simulink model "wahadlo"  (R2021b)
settings: Solver=ode45  StartTime=0.0  StopTime=10.0  RelTol=1e-3  EnableMultiTasking=on
settings Model: Creator=Student  LastModifiedBy=adria
settings SolverCC: AlgebraicLoopSolver=TrustRegion
settings DataIOCC: LimitDataPoints=on  SaveFormat=Array  SignalLoggingSaveFormat=ModelDataLogs  ReturnWorkspaceOutputs=off  SignalLoggingName=sigsOut
settings OptimizationCC: ExpressionDepthLimit=2147483647  InitFltsAndDblsToZero=on  LifeSpan=inf
settings DebuggingCC: SaveWithParameterizedLinksMsg=none  UnderspecifiedInitializationDetection=Classic  MergeDetectMultiDrivingBlocksExec=none  SignalResolutionControl=TryResolveAllWithWarning  MultiTaskDSMMsg=warning  MultiTaskCondExecSysMsg=none  FcnCallInpInsideContextMsg=warning  StateNameClashWarn=warning  SFUnexpectedBacktrackingDiag=warning  SFNoUnconditionalDefaultTransitionDiag=warning  SFExecutionAtInitializationDiag=none  SFMachineParentedDataDiag=warning  ArithmeticOperatorsInVariantConditions=warning
settings HardwareCC: ProdBitPerPointer=32  ProdBitPerSizeT=32  ProdBitPerPtrDiffT=32  ProdLargestAtomicFloat=None  ProdIntDivRoundTo=Undefined  ProdEndianess=Unspecified  ProdWordSize=32  ProdHWDeviceType=32-bit Generic  TargetUnknown=on
settings ModelReferenceCC: PropagateSignalLabelsOutOfModel=off
settings SFSimCC: SimUseLocalCustomCode=off  CustomCodeUndefinedFunction=UseInterfaceOnly
settings RTWCC: RTWUseLocalCustomCode=off
settings CodeAppCC: StateflowObjectComments=on
settings GRTTargetCC: TargetFcnLib=ansi_tfl_tmw.mat  TargetLangStandard=C89/C90 (ANSI)  ModelReferenceCompliant=off  ParMdlRefBuildCompliant=off  CompOptLevelCompliant=off  ConcurrentExecutionCompliant=off  CombineOutputUpdateFcns=off  MatFileLogging=off  MATLABClassNameForMDSCustomization=Simulink.SoftwareTarget.TargetSpecificTriggerConfigurationBase  GRTInterface=on
settings ConfigComp: CovMetricSettings=dw  CovSaveCumulativeToWorkspaceVar=on  CovSaveSingleToWorkspaceVar=on  CovExternalEMLEnable=off

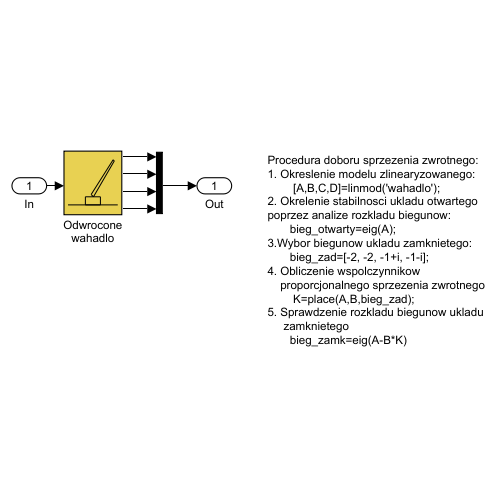
[thumbnail: Simulink's stored preview of the top-level diagram]
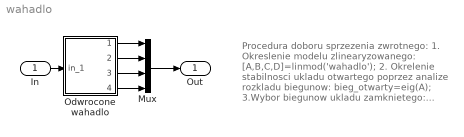
== system wahadlo ==
  note: Procedura doboru sprzezenia zwrotnego:
      | 1. Okreslenie modelu zlinearyzowanego:
      |         [A,B,C,D]=linmod('wahadlo');
      | 2. Okrelenie stabilnosci ukladu otwartego
      | poprzez analize rozkladu biegunow:
      |        bieg_otwarty=eig(A);
      | 3.Wybor biegunow ukladu zamknietego:
      |        bieg_zad=[-2, -2, -1+i, -1-i];
      | 4. Obliczenie wspolczynnikow
      |     proporcjonalnego sprzezenia zwrotnego
      |         K=place(A,B,bieg_zad);
      | 5. Sprawdzenie rozkladu biegunow ukladu
      |      zamknietego
      |        bieg_zamk=eig(A-B*K)
  In : Inport
  Mux : Mux
  Odwrocone wahadlo : Subsystem  mask(Odwrocone wahadlo){init_cond=[0  0  0  0], specs=[8         0.1           1         9.8]}
      mask prompts: init_cond "Poczatkowe(kat, predkosc katowa, pozycja wozka,  predkosc wozka):"; specs "Parametry (dlugosc, masa wahadla, masa wozka, g):"
      mask help: Odwrocone wahadlo
      mask init:
      | l=specs(1)/2;m=specs(2);mc=specs(3);g=specs(4);
      mask Help: Odwrocone wahadlo
      mask Display: plot(-4,-1,4,6,[0 3 2.8 -0.2 0],[1 5 5.15 1.15 1],[-1 -1 1 1 -1],[1 0 0 1 1],[-3.5 3.5],[0 0])
  Out : Outport  VectorParamsAs1DForOutWhenUnconnected=off
  wires:
  In/1 -> Odwrocone wahadlo/1(in_1)
  Odwrocone wahadlo/1(out_1) -> Mux/1
  Odwrocone wahadlo/2(out_2) -> Mux/2
  Odwrocone wahadlo/3(out_3) -> Mux/3
  Odwrocone wahadlo/4(out_4) -> Mux/4
  Mux/1 -> Out/1

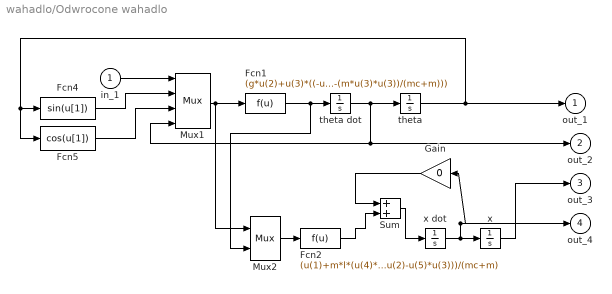
== system wahadlo/Odwrocone wahadlo ==
  in_1 : Inport
  Fcn1 : Fcn  Expr=(g*u(2)+u(3)*((-u(1)-m*l*u(4)*u(4)*u(2))/(mc+m)))/(l*(4/3-(m*u(3)*u(3))/(mc+m)))
  Fcn2 : Fcn  Expr=(u(1)+m*l*(u(4)*u(4)*u(2)-u(5)*u(3)))/(mc+m)
  Fcn4 : Fcn
  Fcn5 : Fcn  Expr=cos(u[1])
  Gain : Gain  Gain=0  SaturateOnIntegerOverflow=on  OutDataTypeStr=Inherit: Same as input  ParamDataTypeStr=Inherit: Same as input
  Mux1 : Mux
  Mux2 : Mux  Inputs=[4,1]
  Sum : Sum  SaturateOnIntegerOverflow=on
  theta : Integrator  InitialCondition=init_cond(1)
  theta dot : Integrator  InitialCondition=init_cond(2)
  x : Integrator  InitialCondition=init_cond(3)
  x dot : Integrator  InitialCondition=init_cond(4)
  out_1 : Outport  InitialOutput=0  VectorParamsAs1DForOutWhenUnconnected=off
  out_2 : Outport  Port=2  InitialOutput=0  VectorParamsAs1DForOutWhenUnconnected=off
  out_3 : Outport  Port=3  InitialOutput=0  VectorParamsAs1DForOutWhenUnconnected=off
  out_4 : Outport  Port=4  InitialOutput=0  VectorParamsAs1DForOutWhenUnconnected=off
  wires:
  in_1/1 -> Mux1/1
  x/1 -> out_3/1
  x dot/1 -> x/1, out_4/1, Gain/1
  Mux1/1 -> Fcn1/1, Mux2/1
  Mux2/1 -> Fcn2/1
  Fcn1/1 -> Mux2/2, theta dot/1
  theta dot/1 -> Mux1/4, out_2/1, theta/1
  Fcn4/1 -> Mux1/2
  Fcn5/1 -> Mux1/3
  theta/1 -> Fcn4/1, Fcn5/1, out_1/1
  Sum/1 -> x dot/1
  Fcn2/1 -> Sum/2
  Gain/1 -> Sum/1
